simulink model "simulinkquestao1"  (R2020a)
settings: Solver=FixedStepAuto  StartTime=0.0  StopTime=1  FixedStep=1e-4  RelTol=1e-3
settings Model: Creator=Dylan  LastModifiedBy=Dylan

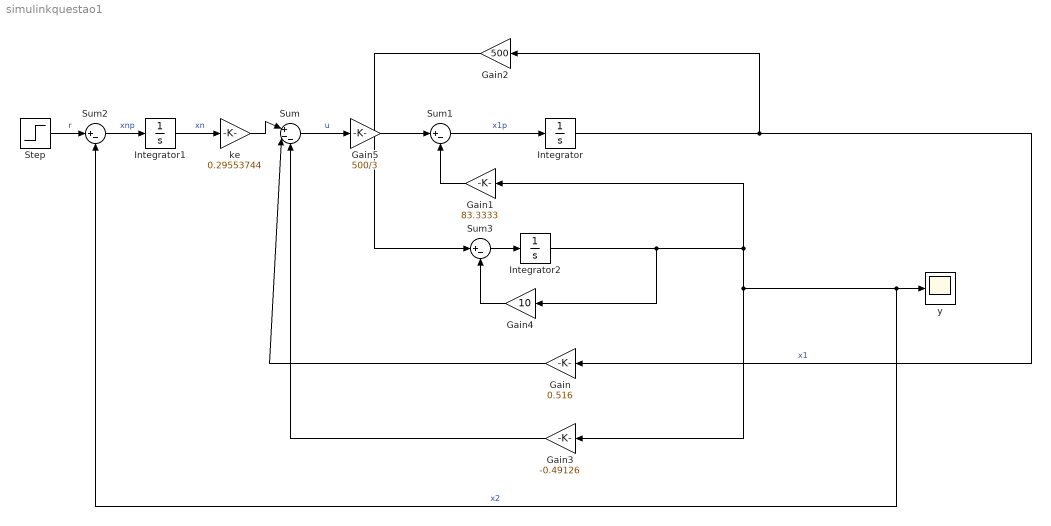
== system simulinkquestao1 ==
  Gain : Gain  Gain=0.516
  Gain1 : Gain  Gain=83.3333
  Gain2 : Gain  Gain=500
  Gain3 : Gain  Gain=-0.49126
  Gain4 : Gain  Gain=10
  Gain5 : Gain  Gain=500/3
  Integrator : Integrator
  Integrator1 : Integrator
  Integrator2 : Integrator
  Step : Step  Time=0  SampleTime=0
  Sum : Sum  Inputs=|+--
  Sum1 : Sum  Inputs=|+-
  Sum2 : Sum  Inputs=|+-
  Sum3 : Sum  Inputs=|+-
  ke : Gain  Gain=0.29553744
  y : Scope
  wires:
  ke/1 -> Sum/1
  Step/1 -> Sum2/1  "r"
  Integrator1/1 -> ke/1  "xn"
  Sum2/1 -> Integrator1/1  "xnp"
  Sum1/1 -> Integrator/1  "x1p"
  Gain/1 -> Sum/2
  Sum/1 -> Gain5/1  "u"
  Integrator2/1 -> Gain4/1, Gain3/1, y/1, Sum2/2, Gain1/1  "x2"
  Integrator/1 -> Gain2/1, Gain/1  "x1"
  Gain1/1 -> Sum1/2
  Gain3/1 -> Sum/3
  Sum3/1 -> Integrator2/1
  Gain2/1 -> Sum3/1
  Gain4/1 -> Sum3/2
  Gain5/1 -> Sum1/1
